simulink model "ICEV_powertrain"  (R2021b)
settings: Solver=FixedStepAuto  StartTime=0.0  StopTime=766  FixedStep=0.01  RelTol=1e-3
undefined symbols (not defined in the file): A, C_d, eff_bat, eff_dt, Eff_map, f_rr, g, id, m, magnitude, Max_Torque, mu, P_aux, r_d, rho, Speed, Torque
libraries: simulink x1, slpidlib x1
settings Model: Creator=Admin  LastModifiedBy=Admin

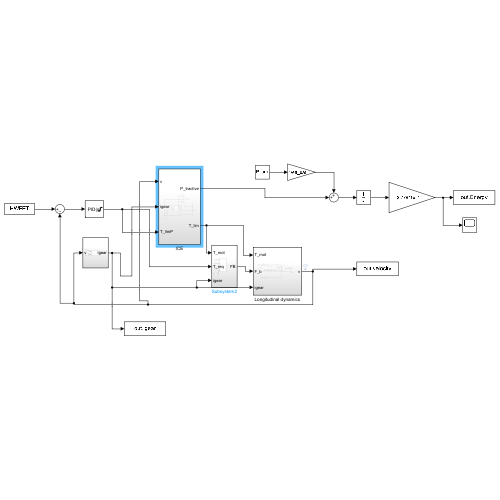
[thumbnail: Simulink's stored preview of the top-level diagram]
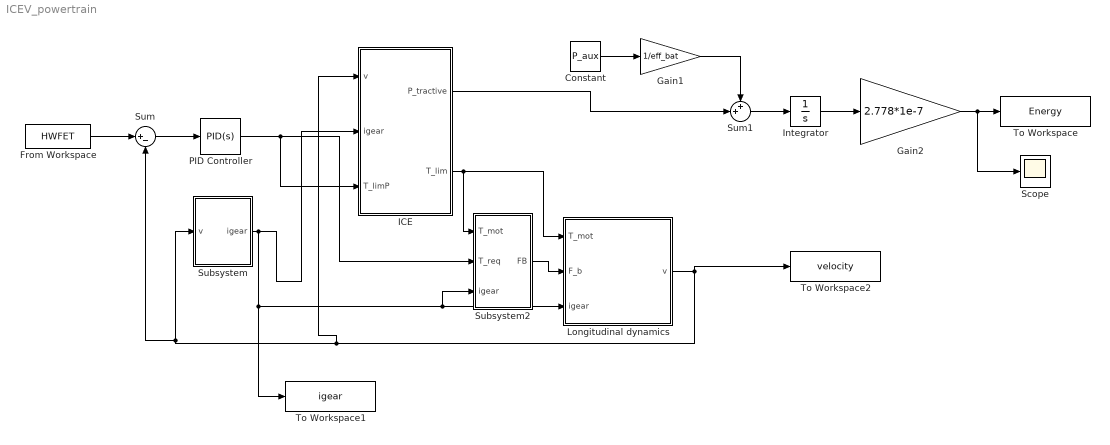
== system ICEV_powertrain ==
  Constant : Constant  Value=P_aux
  From Workspace : FromWorkspace  VariableName=HWFET
  Gain1 : Gain  Gain=1/eff_bat
  Gain2 : Gain  Gain=2.778*1e-7
  ICE : Subsystem
  Integrator : Integrator
  Longitudinal dynamics : Subsystem
  PID Controller : slpidlib/PID Controller  Controller=PID  Form=Parallel  TimeDomain=Continuous-time  UseExternalTs=off  SampleTime=-1  IntegratorMethod=Forward Euler  FilterMethod=Forward Euler  ControllerParametersSource=internal  P=300  I=0  D=0  UseFilter=on  N=100  TunerSelectOption=Transfer Function Based (PID Tuner App)  InitialConditionSource=internal  InitialConditionForIntegrator=0  InitialConditionForFilter=0  DifferentiatorICPrevScaledInput=0  ExternalReset=none  TrackingMode=off  Kt=1  LimitOutput=on  SatLimitsSource=internal  UpperSaturationLimit=inf  LowerSaturationLimit=-m*g*mu  LinearizeAsGain=on  AntiWindupMode=none  Kb=1  POutMin=[]  POutMax=[]  IOutMin=[]  IOutMax=[]  DOutMin=[]  DOutMax=[]  NOutMin=[]  NOutMax=[]  SumOutMin=[]  SumOutMax=[]  SaturationOutMin=[]  SaturationOutMax=[]  PParamMin=[]  PParamMax=[]  IParamMin=[]  IParamMax=[]  DParamMin=[]  DParamMax=[]  NParamMin=[]  NParamMax=[]  KbParamMin=[]  KbParamMax=[]  KtParamMin=[]  KtParamMax=[]  KbOutMin=[]  KbOutMax=[]  KtOutMin=[]  KtOutMax=[]  IntegratorOutMin=[]  IntegratorOutMax=[]  FilterOutMin=[]  FilterOutMax=[]  SumI1OutMin=[]  SumI1OutMax=[]  SumI2OutMin=[]  SumI2OutMax=[]  SumI3OutMin=[]  SumI3OutMax=[]  SumI4OutMin=[]  SumI4OutMax=[]  SumDOutMin=[]  SumDOutMax=[]  DifferentiatorOutMin=[]  DifferentiatorOutMax=[]  FilterDiffOutCoefMin=[]  FilterDiffOutCoefMax=[]  ReciprocalOutMin=[]  ReciprocalOutMax=[]  SumDenOutMin=[]  SumDenOutMax=[]  SumNumOutMin=[]  SumNumOutMax=[]  DivideOutMin=[]  DivideOutMax=[]  UdiffTsProdOutMin=[]  UdiffTsProdOutMax=[]  NTsProdOutMin=[]  NTsProdOutMax=[]  UintegralTsProdOutMin=[]  UintegralTsProdOutMax=[]  UngainTsProdOutMin=[]  UngainTsProdOutMax=[]  IntegratorContinuousStateAttributes=''  IntegratorStateMustResolveToSignalObject=off  IntegratorRTWStateStorageClass=Auto  FilterContinuousStateAttributes=''  FilterStateMustResolveToSignalObject=off  FilterRTWStateStorageClass=Auto  ParallelPVariant=InternalParameters  IdealPVariant=Disabled  IVariant=InternalParameters  DVariant=InternalParameters  IntegratorVariant=Continuous  SatVariant=Enabled  AWVariant=Passthrough  PCopyVariant=Disabled  TRVariant=Disabled  FdbkBlocksVariant=Forward  IdealPFdbkVariant=Disabled  SatFdbkVariant=Disabled  DerivativeFilterVariant=ContFilter  NVariant=InternalParameters  NCopyVariant=Disabled  FilterICVariant=InternalICsFilter  IntegratorICVariant=InternalICs  ExternalResetVariant=Disabled  TRSumVariant=Passthrough  SumFdbkVariant=Disabled  SumVariant=Sum_PID  TsampFilterVariant=InternalTs  TsampNgainVariant=Passthrough  TsampIntegralVariant=Passthrough  ExternalSaturationOutDataTypeStr=Inherit: Same as second input
  Scope : Scope
  Subsystem : Subsystem
  Subsystem2 : Subsystem
  Sum : Sum  Inputs=|+-
  Sum1 : Sum  Inputs=++|
  To Workspace : ToWorkspace  VariableName=Energy  SaveFormat=Timeseries  SampleTime=-1
  To Workspace1 : ToWorkspace  VariableName=igear  SaveFormat=Timeseries  SampleTime=-1
  To Workspace2 : ToWorkspace  VariableName=velocity  SaveFormat=Timeseries  SampleTime=-1
  wires:
  From Workspace/1 -> Sum/1
  Sum/1 -> PID Controller/1
  Subsystem/1(igear) -> To Workspace1/1, Subsystem2/3(igear), Longitudinal dynamics/3(igear), ICE/2(igear)
  Constant/1 -> Gain1/1
  Gain1/1 -> Sum1/1
  Sum1/1 -> Integrator/1
  Integrator/1 -> Gain2/1
  Gain2/1 -> Scope/1, To Workspace/1
  PID Controller/1 -> Subsystem2/2(T_req), ICE/3(T_limP)
  ICE/1(P_tractive) -> Sum1/2
  Longitudinal dynamics/1(v) -> To Workspace2/1, ICE/1(v), Sum/2, Subsystem/1(v)
  ICE/2(T_lim) -> Subsystem2/1(T_mot), Longitudinal dynamics/1(T_mot)
  Subsystem2/1(FB) -> Longitudinal dynamics/2(F_b)

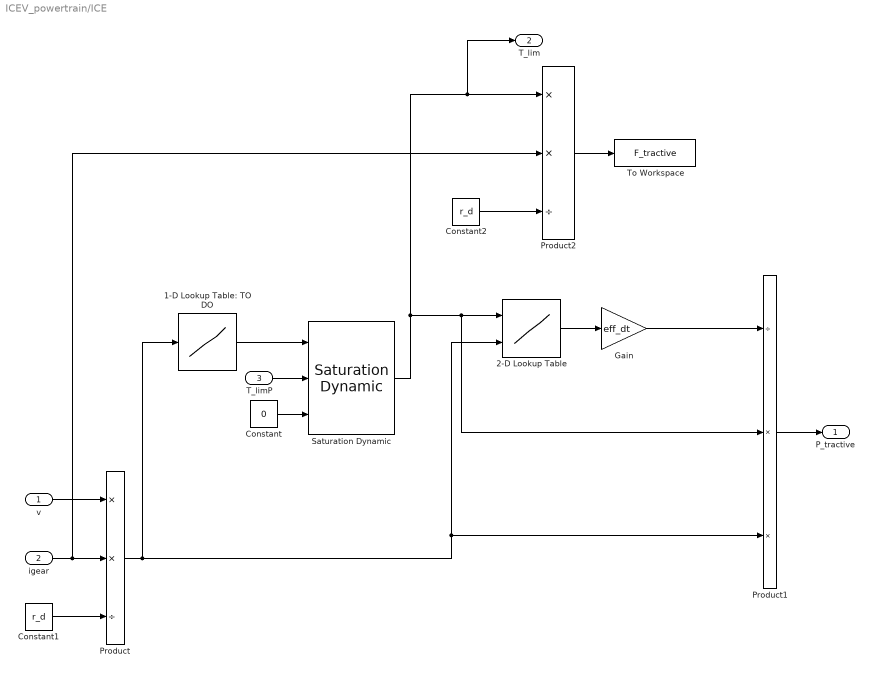
== system ICEV_powertrain/ICE ==
  v : Inport
  igear : Inport  Port=2
  T_limP : Inport  Port=3
  "1-D Lookup Table: TO DO " : Lookup_n-D  NumberOfTableDimensions=1  BreakpointsForDimension1=Speed  Table=Max_Torque  InternalRulePriority=Speed  RndMeth=Simplest  InputSameDT=on
  2-D Lookup Table : Lookup_n-D  BreakpointsForDimension1=Torque  BreakpointsForDimension2=Speed  Table=Eff_map  InternalRulePriority=Speed  RndMeth=Simplest  InputSameDT=on
      settings: InputPortMap=u0,u1
  Constant : Constant  Value=0
  Constant1 : Constant  Value=r_d
  Constant2 : Constant  Value=r_d
  Gain : Gain  Gain=eff_dt
  Product : Product  Inputs=**/
  Product1 : Product  Inputs=/**
  Product2 : Product  Inputs=**/
  Saturation Dynamic : simulink/Discontinuities/Saturation Dynamic  OutMin=[]  OutMax=[]  OutDataTypeStr=Inherit: Same as second input  OutDataType=fixdt(1, 16)  OutScaling=2^-10  DoSatur=off
  To Workspace : ToWorkspace  VariableName=F_tractive  SaveFormat=Timeseries  SampleTime=-1
  P_tractive : Outport
  T_lim : Outport  Port=2
  wires:
  v/1 -> Product/1
  igear/1 -> Product2/2, Product/2
  Constant1/1 -> Product/3
  Product/1 -> "1-D Lookup Table: TO DO "/1, 2-D Lookup Table/2, Product1/3
  Gain/1 -> Product1/1
  Constant/1 -> Saturation Dynamic/3
  T_limP/1 -> Saturation Dynamic/2
  "1-D Lookup Table: TO DO "/1 -> Saturation Dynamic/1
  2-D Lookup Table/1 -> Gain/1
  Constant2/1 -> Product2/3
  Saturation Dynamic/1 -> Product1/2, 2-D Lookup Table/1, T_lim/1, Product2/1
  Product2/1 -> To Workspace/1
  Product1/1 -> P_tractive/1

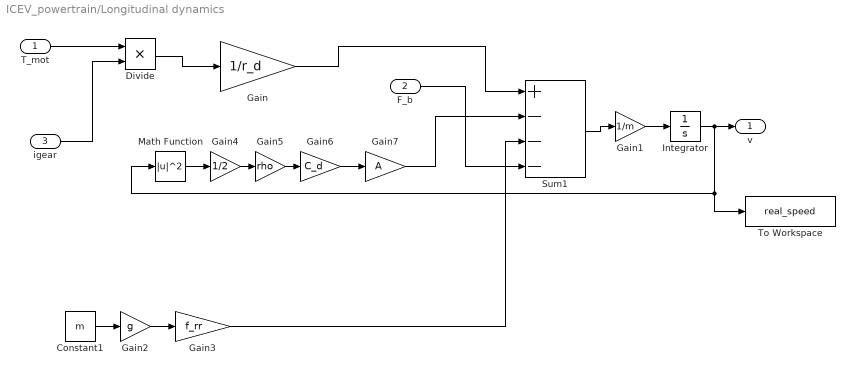
== system ICEV_powertrain/Longitudinal dynamics ==
  T_mot : Inport
  F_b : Inport  Port=2
  igear : Inport  Port=3
  Constant1 : Constant  Value=m
  Divide : Product  Inputs=**
  Gain : Gain  Gain=1/r_d
  Gain1 : Gain  Gain=1/m
  Gain2 : Gain  Gain=g
  Gain3 : Gain  Gain=f_rr
  Gain4 : Gain  Gain=1/2
  Gain5 : Gain  Gain=rho
  Gain6 : Gain  Gain=C_d
  Gain7 : Gain  Gain=A
  Integrator : Integrator
  Math Function : Math  Operator=magnitude^2  SaturateOnIntegerOverflow=on
  Sum1 : Sum  Inputs=+---
  To Workspace : ToWorkspace  VariableName=real_speed  SaveFormat=Timeseries  SampleTime=-1
  v : Outport
  wires:
  T_mot/1 -> Divide/1
  Gain7/1 -> Sum1/2
  Sum1/1 -> Gain1/1
  Gain1/1 -> Integrator/1
  Integrator/1 -> Math Function/1, To Workspace/1, v/1
  Gain/1 -> Sum1/1
  igear/1 -> Divide/2
  Divide/1 -> Gain/1
  Constant1/1 -> Gain2/1
  Gain2/1 -> Gain3/1
  Gain3/1 -> Sum1/3
  F_b/1 -> Sum1/4
  Gain5/1 -> Gain6/1
  Gain6/1 -> Gain7/1
  Gain4/1 -> Gain5/1
  Math Function/1 -> Gain4/1

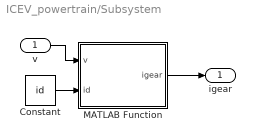
== system ICEV_powertrain/Subsystem ==
  v : Inport
  Constant : Constant  Value=id
  MATLAB Function : MATLAB Function  TreatAsAtomicUnit=on
  igear : Outport
  wires:
  MATLAB Function/1(igear) -> igear/1
  v/1 -> MATLAB Function/1(v)
  Constant/1 -> MATLAB Function/2(id)

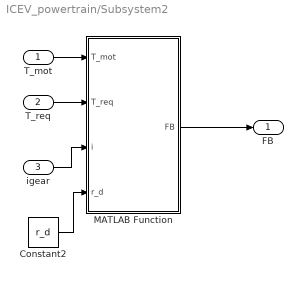
== system ICEV_powertrain/Subsystem2 ==
  T_mot : Inport
  T_req : Inport  Port=2
  igear : Inport  Port=3
  Constant2 : Constant  Value=r_d
  MATLAB Function : MATLAB Function  TreatAsAtomicUnit=on
  FB : Outport
  wires:
  MATLAB Function/1(FB) -> FB/1
  Constant2/1 -> MATLAB Function/4(r_d)
  T_req/1 -> MATLAB Function/2(T_req)
  T_mot/1 -> MATLAB Function/1(T_mot)
  igear/1 -> MATLAB Function/3(i)

== matlab function ICEV_powertrain/Subsystem/MATLAB Function ==
  data: v input; igear output; id input
function igear = fcn(v,id)

v1 = v*3.6;

if v1<=10
    igear = 3.07*id;
elseif (v1>10) & (v1<=30)
    igear = 1.77*id;
elseif (v1>30) & (v1<=50)
    igear = 1.19*id;
elseif (v1>50) & (v1<75)
    igear = 0.87*id;
else 
    igear = 0.7*id;
end
end

== matlab function ICEV_powertrain/Subsystem2/MATLAB Function ==
  data: T_mot input; FB output; T_req input; i input; r_d input
function FB = fcn(T_mot,T_req,i,r_d)

if T_req<0 && T_mot>T_req
    FB = (T_mot-T_req)*(i/r_d);
else 
    FB = 0;
end
end
